simulink model "prueba_kalman_filter"  (R2021a)
settings: Solver=VariableStepAuto  StartTime=0.0  StopTime=inf  RelTol=1e-3
undefined symbols (not defined in the file or in its folder): DiscIntNeverNeededParam
libraries: simulink x2, sharedTrackingLibrary x1
settings Model: EnablePacing=on  Creator=xboxk  LastModifiedBy=xboxk

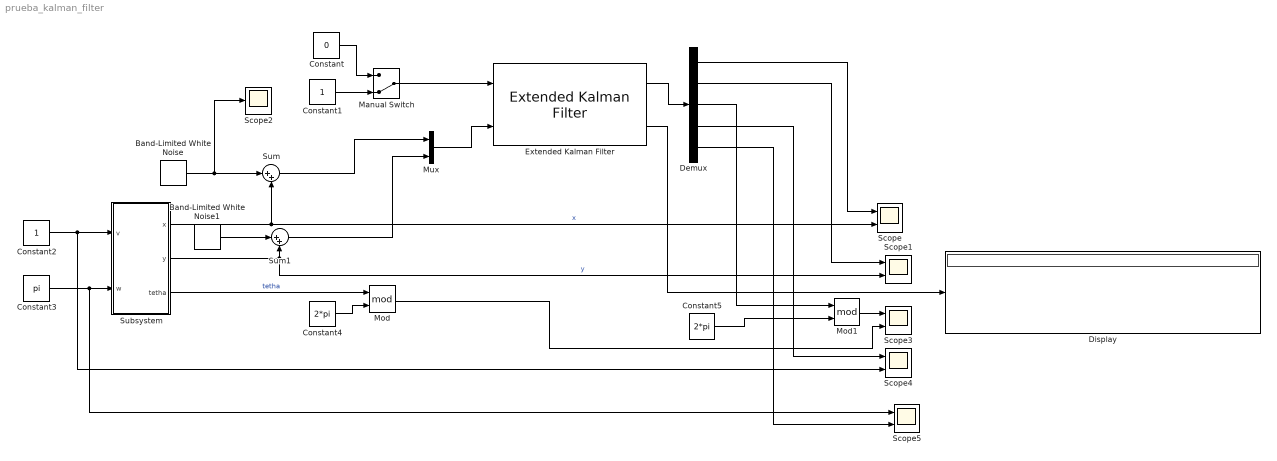
== system prueba_kalman_filter ==
  Band-Limited White Noise : simulink/Sources/Band-Limited White Noise  Cov=[0.00005]  Ts=0.01  seed=[23341]
  Band-Limited White Noise1 : simulink/Sources/Band-Limited White Noise  Cov=[0.00005]  Ts=0.01  seed=[23341]
  Constant : Constant  Value=0
  Constant1 : Constant
  Constant2 : Constant
  Constant3 : Constant  Value=pi
  Constant4 : Constant  Value=2*pi
  Constant5 : Constant  Value=2*pi
  Demux : Demux  Outputs=5
  Display : Display
  Extended Kalman Filter : sharedTrackingLibrary/Extended Kalman Filter  StateTransitionFcn=transitionFcn  HasStateTransitionJacobianFcn=off  StateTransitionJacobianFcn=transitionJacobianFcn  HasAdditiveProcessNoise=Additive  ProcessNoise=diag([0.01,0.001,0.001,0.001,0.001])  HasTimeVaryingProcessNoise=off  HasStateTransitionFcnExtraArgument=0  InitialState=[0,0,0,1,pi]  InitialStateCovariance=diag([1,1,1,1,1])  MeasurementFcn1=myMeasurementFcn  HasMeasurementJacobianFcn1=off  HasMeasurementEnablePort1=on  HasAdditiveMeasurementNoise1=Additive  MeasurementNoise1=diag([0.5,0.5])  HasTimeVaryingMeasurementNoise1=off  HasMeasurementFcnExtraArgument1=0  MeasurementFcn2=myMeasurementFcn  HasMeasurementJacobianFcn2=off  HasMeasurementEnablePort2=off  HasAdditiveMeasurementNoise2=Additive  MeasurementNoise2=1  HasTimeVaryingMeasurementNoise2=off  HasMeasurementFcnExtraArgument2=0  MeasurementFcn3=myMeasurementFcn  HasMeasurementJacobianFcn3=off  HasMeasurementEnablePort3=off  HasAdditiveMeasurementNoise3=Additive  MeasurementNoise3=1  HasTimeVaryingMeasurementNoise3=off  HasMeasurementFcnExtraArgument3=0  MeasurementFcn4=myMeasurementFcn  HasMeasurementJacobianFcn4=off  HasMeasurementEnablePort4=off  HasAdditiveMeasurementNoise4=Additive  MeasurementNoise4=1  HasTimeVaryingMeasurementNoise4=off  HasMeasurementFcnExtraArgument4=0  MeasurementFcn5=myMeasurementFcn  HasMeasurementJacobianFcn5=off  HasMeasurementEnablePort5=off  HasAdditiveMeasurementNoise5=Additive  MeasurementNoise5=1  HasTimeVaryingMeasurementNoise5=off  HasMeasurementFcnExtraArgument5=0  EnableMultirate=off  StateTransitionFcnSampleTime=1  MeasurementFcn1SampleTime=1  MeasurementFcn2SampleTime=1  MeasurementFcn3SampleTime=1  MeasurementFcn4SampleTime=1  MeasurementFcn5SampleTime=1  UseCurrentEstimator=on  OutputStateCovariance=on  DataType=double  SampleTime=0.01  NumberOfMeasurements=1
      settings: SourceProductBaseCode=CT,DR,TF,ID,LP,NV,AR,RO,RR,UV,VE
  Manual Switch : ManualSwitch  CurrentSetting=0
  Mod : Math  Operator=mod  SaturateOnIntegerOverflow=on
  Mod1 : Math  Operator=mod  SaturateOnIntegerOverflow=on
  Mux : Mux  Inputs=2
  Scope{,1,3..5} (5 alike) : Scope  NumInputPorts=2
  Scope2 : Scope
  Subsystem : Subsystem  mask{pos_ini_x=0, pos_ini_y=0, pos_ini_w=0, sample_time=0.01}
      mask prompts: pos_ini_x "Posicion inicial x:"; pos_ini_y "Posicion inicial y:"; pos_ini_w "Posicion inicial w:"; sample_time "Sample time:"
      mask help: Este bloque recibira los valores de velocidad y velocidad angular, y saldran los valores de la posicion en x,y y la orientacion tetha.
  Sum : Sum  Inputs=|++
  Sum1 : Sum  Inputs=|++
  wires:
  Constant/1 -> Manual Switch/1
  Constant1/1 -> Manual Switch/2
  Manual Switch/1 -> Extended Kalman Filter/1
  Constant2/1 -> Scope4/2, Subsystem/1(v)
  Constant3/1 -> Scope5/1, Subsystem/2(w)
  Mux/1 -> Extended Kalman Filter/2
  Band-Limited White Noise/1 -> Scope2/1, Sum/1
  Subsystem/1(x) -> Sum/2, Scope/2  "x"
  Band-Limited White Noise1/1 -> Sum1/1
  Subsystem/2(y) -> Scope1/2, Sum1/2  "y"
  Sum/1 -> Mux/1
  Sum1/1 -> Mux/2
  Extended Kalman Filter/1 -> Demux/1
  Demux/1 -> Scope/1
  Demux/2 -> Scope1/1
  Demux/4 -> Scope4/1
  Demux/5 -> Scope5/2
  Subsystem/3(tetha) -> Mod/1  "tetha"
  Mod/1 -> Scope3/2
  Constant4/1 -> Mod/2
  Extended Kalman Filter/2 -> Display/1
  Mod1/1 -> Scope3/1
  Demux/3 -> Mod1/1
  Constant5/1 -> Mod1/2

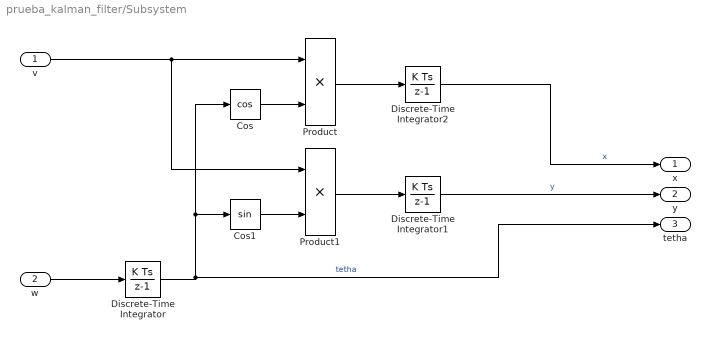
== system prueba_kalman_filter/Subsystem ==
  v : Inport
  w : Inport  Port=2
  Cos : Trigonometry  Operator=cos
  Cos1 : Trigonometry
  Discrete-Time Integrator : DiscreteIntegrator  InitialCondition=pos_ini_w  SampleTime=sample_time  ICPrevOutput=DiscIntNeverNeededParam  ICPrevScaledInput=DiscIntNeverNeededParam
  Discrete-Time Integrator1 : DiscreteIntegrator  InitialCondition=pos_ini_y  SampleTime=sample_time  ICPrevOutput=DiscIntNeverNeededParam  ICPrevScaledInput=DiscIntNeverNeededParam
  Discrete-Time Integrator2 : DiscreteIntegrator  InitialCondition=pos_ini_x  SampleTime=sample_time  ICPrevOutput=DiscIntNeverNeededParam  ICPrevScaledInput=DiscIntNeverNeededParam
  Product : Product
  Product1 : Product
  x : Outport
  y : Outport  Port=2
  tetha : Outport  Port=3
  wires:
  v/1 -> Product1/1, Product/1
  Cos/1 -> Product/2
  w/1 -> Discrete-Time Integrator/1
  Product/1 -> Discrete-Time Integrator2/1
  Product1/1 -> Discrete-Time Integrator1/1
  Discrete-Time Integrator/1 -> tetha/1, Cos/1, Cos1/1  "tetha"
  Discrete-Time Integrator1/1 -> y/1  "y"
  Cos1/1 -> Product1/2
  Discrete-Time Integrator2/1 -> x/1  "x"
